simulink model "hp_memristor"  (Simulink 8.3)
settings: Solver=ode45  StartTime=0.0  StopTime=0.01  RelTol=1e-3
values from neighbouring files (symbols this model uses):
  D = 1e-8    (= 1e-08)    [test_hp_memristor.m]    (also in test_memristor.m)
  muv = 1e-11    [test_hp_memristor.m]    (also in test_memristor.m)
  Rinit = 11e3    (= 11000)    [test_hp_memristor.m]    (also in test_memristor.m)
  Roff = 16e3    (= 16000)    [test_hp_memristor.m]    (also in test_memristor.m)
  Ron = 100    [test_hp_memristor.m]    (also in test_memristor.m)
  v_amp = 10    [test_hp_memristor.m]    (also in test_memristor.m)
  vth = 30    [test_IM_neuron.m]    (also in test_hp_memristor.m = 0; test_memristor.m = 0)
  win_type = 2    [test_hp_memristor.m]    (also in test_memristor.m)
settings Model: Creator=wjj  LastModifiedBy=wjj
settings DataIOCC: SignalLoggingSaveFormat=Dataset
settings DebuggingCC: UnderspecifiedInitializationDetection=Simplified  StateNameClashWarn=none
settings GRTTargetCC: CombineOutputUpdateFcns=on  GRTInterface=off

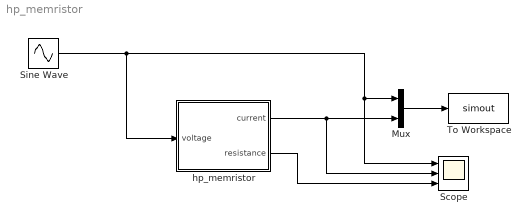
== system hp_memristor ==
  Mux : Mux  Inputs=2
  Scope : Scope  NumInputPorts=3
      settings: YMin=-0.00015~2500~-1.5  YMax=0.00015~12500~1.5
  Sine Wave : Sin  Amplitude=v_amp  Frequency=1e3*2*pi  SampleTime=1e-5
  To Workspace : ToWorkspace  VariableName=simout  SampleTime=1e-5
      settings: Save2DSignal=2-D array (concatenate along first dimension)
  hp_memristor : Subsystem  mask{vth=vth, muv=muv, D=D, Ron=Ron, Roff=Roff, Rinit=Rinit, win_type=win_type}
      mask prompts: win_type "Windows Function Type"
  wires:
  Sine Wave/1 -> Mux/1, Scope/1, hp_memristor/1(voltage)
  Mux/1 -> To Workspace/1
  hp_memristor/1(current) -> Scope/2, Mux/2
  hp_memristor/2(resistance) -> Scope/3

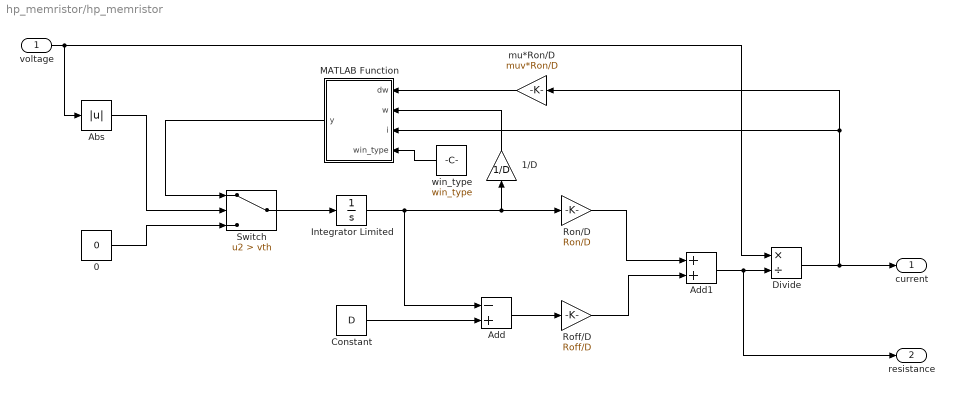
== system hp_memristor/hp_memristor ==
  voltage : Inport
  0 : Constant  Value=0
  1/D : Gain  Gain=1/D
  Abs : Abs
  Add : Sum  Inputs=-+
  Add1 : Sum
  Constant : Constant  Value=D
  Divide : Product  Inputs=*/
  Integrator Limited : Integrator  InitialCondition=(Roff- Rinit)/(Roff - Ron)*D  LimitOutput=on  UpperSaturationLimit=D  LowerSaturationLimit=0
  MATLAB Function : MATLAB Function  TreatAsAtomicUnit=on
  Roff/D : Gain  Gain=Roff/D
  Ron/D : Gain  Gain=Ron/D
  Switch : Switch  Criteria=u2 > Threshold  Threshold=vth
  mu*Ron/D : Gain  Gain=muv*Ron/D
  win_type : Constant  Value=win_type
  current : Outport
  resistance : Outport  Port=2
  wires:
  voltage/1 -> Abs/1, Divide/1
  Ron/D/1 -> Add1/1
  Constant/1 -> Add/2
  Add/1 -> Roff/D/1
  Integrator Limited/1 -> Add/1, Ron/D/1, 1/D/1
  Roff/D/1 -> Add1/2
  Add1/1 -> resistance/1, Divide/2
  Divide/1 -> current/1, mu*Ron/D/1, MATLAB Function/3(i)
  mu*Ron/D/1 -> MATLAB Function/1(dw)
  win_type/1 -> MATLAB Function/4(win_type)
  1/D/1 -> MATLAB Function/2(w)
  Abs/1 -> Switch/2
  MATLAB Function/1(y) -> Switch/1
  0/1 -> Switch/3
  Switch/1 -> Integrator Limited/1

== matlab function hp_memristor/MATLAB Function ==
  data: dw input double; y output double; w input double; i input double; win_type input double
function y = windows_fun(dw, w, i,win_type)

    
if win_type == 1
    y = dw*(1 - 4*(0.5-w)^2);
elseif win_type == 2
    fix_w = (0.5 - w)*tanh(i);
    if fix_w > 0
        y = dw*(1 - 4*(0.5-w)^2 + fix_w);
    else
        y = dw*(1 - 4*(0.5-w)^2);
    end
else 
    y = dw;
end

end
